simulink model "GFM_L_Filter_vc"  (R2019b)
settings: Solver=ode23tb  StartTime=0.0  StopTime=Simulation_Time  FixedStep=Time_Step2  MaxStep=1e-5  RelTol=1e-3
PreLoadFcn:
  | GFM_L_Filter_Init;
InitFcn:
  | GFM_L_Filter_Init;
undefined symbols (not defined in the file): Chosen_Strategy, DiscIntNeverNeededParam, dur1, dur2, egfault, fb, GRD00_Lg, GRD00_Lg2, GRD00_Rg, GRD00_Rg2, Ib2, Kc, kd, Ki_cc_cp, Ki_Inertia_Less, Kp_cc_cp, kp_GFo, Kp_Inertia_Less, R, Sb, SimStart, Theta_Vvsc0, Time_Step, Time_Step2, Ug, Va0, Vb0, Vb1, Vb2, Vc0, Vm0, VSC01_id0, Vvsc0, wb, Zb
libraries: powerlib x30, Control_Lib x15, simulink x7, Source_Lib x1, powerlib_meascontrol x1
(part 2 of 2)

== system GFM_L_Filter_vc/Generic Voltage Source/Source_For_OP ==
  v_abc_ref : Inport
  Controlled Voltage Source1 : powerlib/Electrical Sources/Controlled Voltage Source  Initialize=off  Source_Type=AC  Amplitude=V0*Ub*sqrt(2/3)*sin(Theta0)  Phase=(Theta0*180/pi)  Frequency=fb  Measurements=None
  Controlled Voltage Source2 : powerlib/Electrical Sources/Controlled Voltage Source  Initialize=off  Source_Type=AC  Amplitude=V0*Ub*sqrt(2/3)*sin(Theta0-2*pi/3)  Phase=(Theta0*180/pi)-120  Frequency=fb  Measurements=None
  Controlled Voltage Source3 : powerlib/Electrical Sources/Controlled Voltage Source  Initialize=off  Source_Type=AC  Amplitude=V0*Ub*sqrt(2/3)*sin(Theta0-4*pi/3)  Phase=(Theta0*180/pi)+120  Frequency=fb  Measurements=None
  Demux : Demux  Outputs=3
  Step : Step  Time=1e-9  SampleTime=0
  Subsystem3 : Subsystem
  Three-Phase Source1 : powerlib/Electrical Sources/Three-Phase Source  InternalConnection=Yn  VoltagePhases=off  Voltage=V0*Ub  PhaseAngle=Theta0  Voltage_phases=[25e3 25e3 25e3]/sqrt(3)  PhaseAngles_phases=[0 -120 +120]  Frequency=fb  NonIdealSource=off  SpecifyImpedance=off  Resistance=0.8929  Inductance=16.58e-3  ShortCircuitLevel=100e6  BaseVoltage=25e3  XRratio=7  BusType=swing  Pref=10e3  Qref=0  Prefabc=[10e3, 10e3, 10e3]  Qrefabc=[0, 0, 0]  Qmin=-inf  Qmax=inf
  A : PMIOPort  Side=Right
  B : PMIOPort  Port=2  Side=Right
  C : PMIOPort  Port=3  Side=Right
  N : PMIOPort  Port=4  Side=Left
  wires:
  Demux/2 -> Controlled Voltage Source2/1
  v_abc_ref/1 -> Demux/1
  Demux/1 -> Controlled Voltage Source1/1
  Demux/3 -> Controlled Voltage Source3/1
  Step/1 -> Subsystem3/1(switch)
  connections:
  Controlled Voltage Source3/LConn1 -- Three-Phase Source1/LConn1 -- N/RConn1 -- Controlled Voltage Source2/LConn1 -- Controlled Voltage Source1/LConn1
  Subsystem3/RConn1 -- A/RConn1
  Subsystem3/RConn2 -- B/RConn1
  Subsystem3/RConn3 -- C/RConn1
  Controlled Voltage Source1/RConn1 -- Subsystem3/LConn1
  Controlled Voltage Source2/RConn1 -- Subsystem3/LConn2
  Controlled Voltage Source3/RConn1 -- Subsystem3/LConn3
  Three-Phase Source1/RConn1 -- Subsystem3/LConn4
  Three-Phase Source1/RConn2 -- Subsystem3/LConn5
  Three-Phase Source1/RConn3 -- Subsystem3/LConn6

== system GFM_L_Filter_vc/GFM_VC_newwith_Pvirt IDEAL_VSC/Control loops2/ pu P//Q computation ==
  v_abc_pu : Inport  PortDimensions=3
  i_abc_pu : Inport  Port=2  PortDimensions=3
  Demux : Demux  Outputs=3
      settings: DisplayOption=none
  Mux : Mux  Inputs=3
  Product1 : Product  InputSameDT=on  SaturateOnIntegerOverflow=on  OutDataTypeStr=Inherit: Same as first input
  Product3 : Product  InputSameDT=on  SaturateOnIntegerOverflow=on  OutDataTypeStr=Inherit: Same as first input
  Sum : Sum  Inputs=+-  InputSameDT=on  SaturateOnIntegerOverflow=on  OutDataTypeStr=Inherit: Same as first input
  Sum1 : Sum  Inputs=1  InputSameDT=on  SaturateOnIntegerOverflow=on  OutDataTypeStr=Inherit: Same as first input
  Sum4 : Sum  Inputs=1  InputSameDT=on  SaturateOnIntegerOverflow=on  OutDataTypeStr=Inherit: Same as first input
  Sum5 : Sum  Inputs=+-  InputSameDT=on  SaturateOnIntegerOverflow=on  OutDataTypeStr=Inherit: Same as first input
  Sum6 : Sum  Inputs=+-  InputSameDT=on  SaturateOnIntegerOverflow=on  OutDataTypeStr=Inherit: Same as first input
  pu->V : Gain  Gain=1/sqrt(3)  SaturateOnIntegerOverflow=on  OutDataTypeStr=Inherit: Same as input  ParamDataTypeStr=Inherit: Same as input
  pu->V1 : Gain  Gain=1/3  SaturateOnIntegerOverflow=on  OutDataTypeStr=Inherit: Same as input  ParamDataTypeStr=Inherit: Same as input
  pu->V2 : Gain  Gain=1/3  SaturateOnIntegerOverflow=on  OutDataTypeStr=Inherit: Same as input  ParamDataTypeStr=Inherit: Same as input
  P : Outport  VectorParamsAs1DForOutWhenUnconnected=off
  Q : Outport  Port=2  VectorParamsAs1DForOutWhenUnconnected=off
  wires:
  pu->V2/1 -> Q/1
  pu->V1/1 -> P/1
  Sum1/1 -> pu->V/1
  Product3/1 -> Sum1/1
  Product1/1 -> Sum4/1
  v_abc_pu/1 -> Product1/1, Demux/1
  i_abc_pu/1 -> Product1/2, Product3/2
  Sum4/1 -> pu->V1/1
  Demux/1 -> Sum/1, Sum6/2
  Demux/2 -> Sum/2, Sum5/1
  Demux/3 -> Sum5/2, Sum6/1
  Sum/1 -> Mux/3
  Sum5/1 -> Mux/1
  Sum6/1 -> Mux/2
  Mux/1 -> Product3/1
  pu->V/1 -> pu->V2/1  "Q"

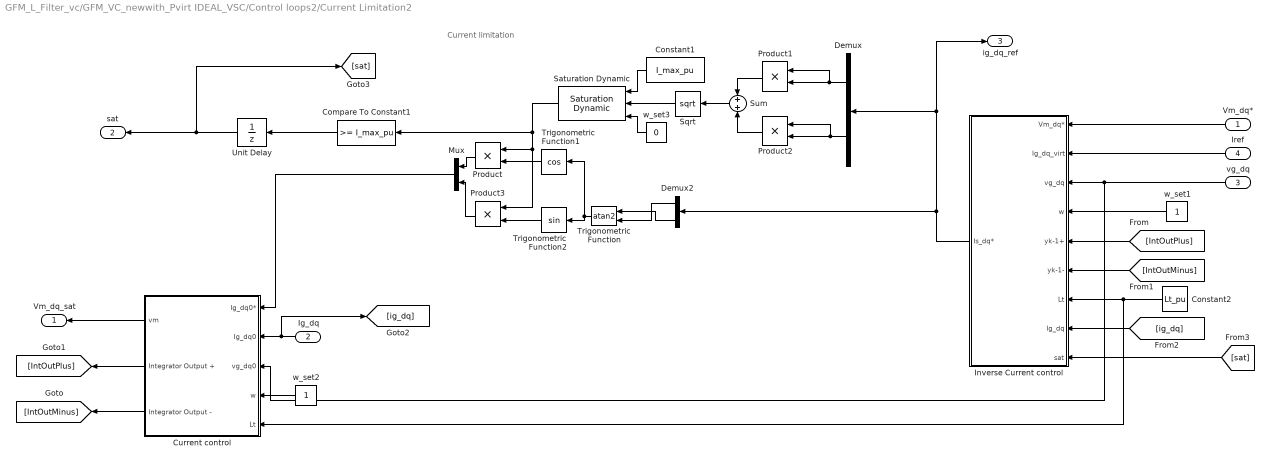
== system GFM_L_Filter_vc/GFM_VC_newwith_Pvirt IDEAL_VSC/Control loops2/Current Limitation2 ==
  note: Current limitation
  Vm_dq* : Inport
  Ig_dq : Inport  Port=2
  vg_dq : Inport  Port=3
  Iref : Inport  Port=4
  Compare To Constant1 : simulink/Logic and Bit Operations/Compare To Constant  relop=>=  const=I_max_pu  OutDataTypeStr=boolean
  Constant1 : Constant  Value=I_max_pu
  Constant2 : Constant  Value=Lt_pu
  Current control : Subsystem
  Demux : Demux  Outputs=2
  Demux2 : Demux  Outputs=2
  Inverse Current control : Subsystem
  Mux : Mux  Inputs=2
  Product{,1..3} (4 alike) : Product
  Saturation Dynamic : simulink/Discontinuities/Saturation Dynamic  OutMin=[]  OutMax=[]  OutDataTypeStr=Inherit: Same as second input  OutDataType=fixdt(1, 16)  OutScaling=2^-10  DoSatur=off
  Sqrt : Sqrt  SaturateOnIntegerOverflow=on
  Sum : Sum
  Trigonometric Function : Trigonometry  Operator=atan2  NumberOfIterations=5  OutputSignalType=real
  Trigonometric Function1 : Trigonometry  Operator=cos
  Trigonometric Function2 : Trigonometry
  Unit Delay : UnitDelay  SampleTime=-1  HasFrameUpgradeWarning=on
  w_set1 : Constant
  w_set2 : Constant
  w_set3 : Constant  Value=0
  Vm_dq_sat : Outport  VectorParamsAs1DForOutWhenUnconnected=off
  sat : Outport  Port=2
  ig_dq_ref : Outport  Port=3
  wires:
  w_set3/1 -> Saturation Dynamic/3
  Product/1 -> Mux/1
  Demux/1 -> Product1/1, Product1/2
  Demux/2 -> Product2/1, Product2/2
  Trigonometric Function2/1 -> Product3/2
  Product2/1 -> Sum/2
  Trigonometric Function1/1 -> Product/2
  Demux2/1 -> Trigonometric Function/2
  Trigonometric Function/1 -> Trigonometric Function2/1, Trigonometric Function1/1
  Product1/1 -> Sum/1
  Sqrt/1 -> Saturation Dynamic/2
  Demux2/2 -> Trigonometric Function/1
  Sum/1 -> Sqrt/1
  Product3/1 -> Mux/2
  Ig_dq/1 -> [ig_dq], Current control/2(Ig_dq0)
  w_set1/1 -> Inverse Current control/4(w)
  w_set2/1 -> Current control/4(w)
  Vm_dq*/1 -> Inverse Current control/1(Vm_dq*)
  Current control/1(vm) -> Vm_dq_sat/1
  Mux/1 -> Current control/1(Ig_dq0*)
  vg_dq/1 -> Current control/3(vg_dq0), Inverse Current control/3(vg_dq)
  Current control/3(Integrator Output -) -> [IntOutMinus]
  [IntOutMinus] -> Inverse Current control/6(yk-1-)
  Current control/2(Integrator Output +) -> [IntOutPlus]
  [IntOutPlus] -> Inverse Current control/5(yk-1+)
  Constant1/1 -> Saturation Dynamic/1
  Saturation Dynamic/1 -> Compare To Constant1/1, Product/1, Product3/1
  Compare To Constant1/1 -> Unit Delay/1
  Constant2/1 -> Current control/5(Lt), Inverse Current control/7(Lt)
  Iref/1 -> Inverse Current control/2(Ig_dq_virt)
  Inverse Current control/1(Is_dq*) -> Demux2/1, ig_dq_ref/1, Demux/1
  [ig_dq] -> Inverse Current control/8(Ig_dq)
  [sat] -> Inverse Current control/9(sat)
  Unit Delay/1 -> [sat], sat/1

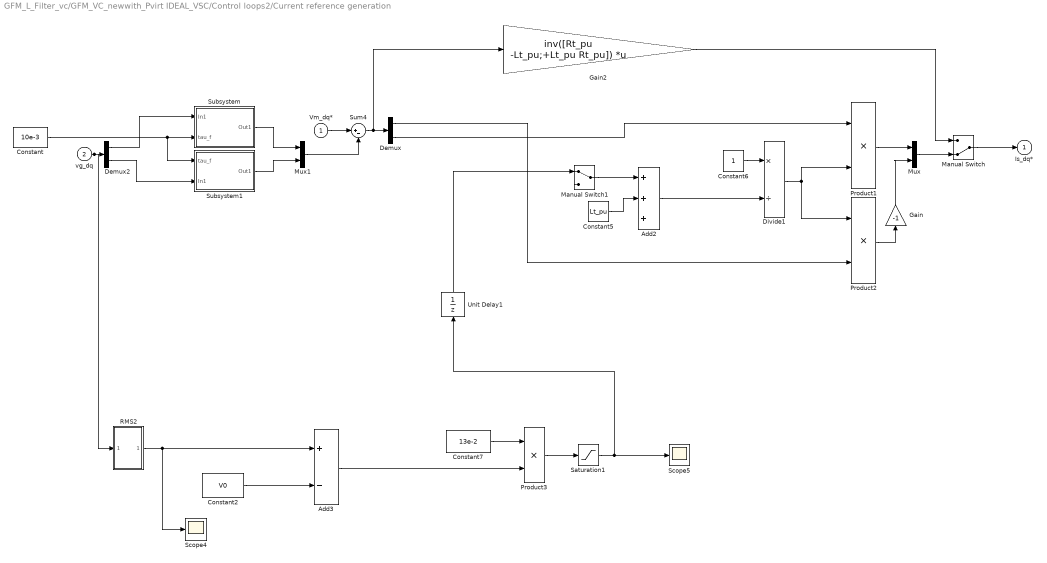
== system GFM_L_Filter_vc/GFM_VC_newwith_Pvirt IDEAL_VSC/Control loops2/Current reference generation ==
  Vm_dq* : Inport
  vg_dq : Inport  Port=2
  Add2 : Sum  Inputs=+++
  Add3 : Sum  Inputs=+-
  Constant : Constant  Value=10e-3
  Constant2 : Constant  Value=V0
  Constant5 : Constant  Value=Lt_pu
  Constant6 : Constant
  Constant7 : Constant  Value=13e-2
  Demux : Demux  Outputs=2
  Demux2 : Demux  Outputs=2
  Divide1 : Product  Inputs=*/
  Gain : Gain  Gain=-1
  Gain2 : Gain  Gain=inv([Rt_pu -Lt_pu;+Lt_pu Rt_pu])  Multiplication=Matrix(K*u)
  Manual Switch : ManualSwitch  CurrentSetting=0
  Manual Switch1 : ManualSwitch
  Mux : Mux  Inputs=2
  Mux1 : Mux  Inputs=2
  Product1 : Product
  Product2 : Product
  Product3 : Product
  RMS2 : Subsystem
  Saturation1 : Saturate  UpperLimit=0  LowerLimit=-0.14
  Scope4 : Scope
  Scope5 : Scope
  Subsystem : Subsystem
  Subsystem1 : Subsystem
  Sum4 : Sum  Inputs=|+-
  Unit Delay1 : UnitDelay  SampleTime=-1  HasFrameUpgradeWarning=on
  Is_dq* : Outport  InitialOutput=0  VectorParamsAs1DForOutWhenUnconnected=off
  wires:
  Unit Delay1/1 -> Manual Switch1/1
  Manual Switch1/1 -> Add2/1
  Vm_dq*/1 -> Sum4/1
  Demux2/2 -> Subsystem1/2(In1)
  Demux2/1 -> Subsystem/1(In1)
  Subsystem/1(Out1) -> Mux1/1
  Subsystem1/1(Out1) -> Mux1/2
  vg_dq/1 -> RMS2/1(Is_dq*), Demux2/1
  Sum4/1 -> Gain2/1, Demux/1
  Mux1/1 -> Sum4/2
  Constant/1 -> Subsystem1/1(tau_f), Subsystem/2(tau_f)
  Demux/2 -> Product1/1
  Product1/1 -> Mux/1
  Product2/1 -> Gain/1
  Demux/1 -> Product2/2
  Manual Switch/1 -> Is_dq*/1
  Gain2/1 -> Manual Switch/1
  Mux/1 -> Manual Switch/2
  Constant5/1 -> Add2/2
  Constant6/1 -> Divide1/1
  Divide1/1 -> Product2/1, Product1/2
  Gain/1 -> Mux/2
  Add2/1 -> Divide1/2
  Product3/1 -> Saturation1/1
  Constant2/1 -> Add3/2
  Constant7/1 -> Product3/1
  Add3/1 -> Product3/2
  RMS2/1(Out1) -> Add3/1, Scope4/1
  Saturation1/1 -> Unit Delay1/1, Scope5/1

== system GFM_L_Filter_vc/GFM_VC_newwith_Pvirt IDEAL_VSC/Control loops2/Power Control Loops1 ==
  P_mes : Inport
  P_set : Inport  Port=2
  delta_PLL : Inport  Port=3
  w_PLL : Inport  Port=4
  sat : Inport  Port=5
  Vg_rms : Inport  Port=6
  Compare To Constant : simulink/Logic and Bit Operations/Compare To Constant  relop===  const=1  OutDataTypeStr=boolean
  Compare To Constant1 : simulink/Logic and Bit Operations/Compare To Constant  relop===  const=2  OutDataTypeStr=boolean
  Compare To Constant2 : simulink/Logic and Bit Operations/Compare To Constant  relop===  const=3  OutDataTypeStr=boolean
  Inertia Less : Subsystem
  Multiport Switch : MultiPortSwitch
  Multiport Switch1 : MultiPortSwitch
  Mux : Mux  Inputs=[1 1]
  PI Controler : Subsystem
  Trigonometric Function : Trigonometry  Operator=cos
  Trigonometric Function1 : Trigonometry
  VSM : Subsystem
  w_set{1..4} (4 alike) : Constant  Value=Chosen_Strategy
  w_set_pu : Constant
  f : Outport  PortDimensions=1  VectorParamsAs1DForOutWhenUnconnected=off
  Theta : Outport  Port=2  VectorParamsAs1DForOutWhenUnconnected=off
  CosSinTheta : Outport  Port=3  PortDimensions=2  VectorParamsAs1DForOutWhenUnconnected=off
  wires:
  Trigonometric Function1/1 -> Mux/2
  Mux/1 -> CosSinTheta/1
  Trigonometric Function/1 -> Mux/1
  Compare To Constant2/1 -> PI Controler/Enable
  Compare To Constant1/1 -> VSM/Enable
  Compare To Constant/1 -> Inertia Less/Enable
  w_set4/1 -> Compare To Constant2/1
  w_set2/1 -> Compare To Constant1/1
  w_set3/1 -> Compare To Constant/1
  Inertia Less/1(frequency) -> Multiport Switch/2
  Multiport Switch/1 -> f/1
  Inertia Less/2(theta) -> Multiport Switch1/2
  VSM/2(theta) -> Multiport Switch1/3
  w_set1/1 -> Multiport Switch/1, Multiport Switch1/1
  VSM/1(frequency) -> Multiport Switch/3
  PI Controler/1(frequency) -> Multiport Switch/4
  PI Controler/2(theta) -> Multiport Switch1/4
  w_set_pu/1 -> PI Controler/3(w_set_pu)
  w_PLL/1 -> Inertia Less/4(w_PLL), VSM/3(w_PLL)
  delta_PLL/1 -> Inertia Less/3(delta_PLL)
  P_set/1 -> Inertia Less/2(P_set), VSM/2(P_set), PI Controler/2(P_set)
  P_mes/1 -> Inertia Less/1(P_mes), VSM/1(P_mes), PI Controler/1(P_mes)
  Multiport Switch1/1 -> Theta/1, Trigonometric Function1/1, Trigonometric Function/1
  sat/1 -> PI Controler/4(sat)
  Vg_rms/1 -> PI Controler/5(Vg_rms)

== system GFM_L_Filter_vc/GFM_VC_newwith_Pvirt IDEAL_VSC/Control loops2/Transient Damping Resistance ==
  ig_dq : Inport
  Filter w_LF : Subsystem
      mask Display: disp('\omega_{LF} / (s + \omega_{LF})','texmode','on')
  Sum5 : Sum  Inputs=|+-
  nq1 : Gain  Gain=Rv
  "Delta_E_dq " : Outport  VectorParamsAs1DForOutWhenUnconnected=off
  wires:
  nq1/1 -> Filter w_LF/1(e), Sum5/2
  Filter w_LF/1(s) -> Sum5/1
  Sum5/1 -> "Delta_E_dq "/1
  ig_dq/1 -> nq1/1

== system GFM_L_Filter_vc/GFM_VC_newwith_Pvirt IDEAL_VSC/Control loops2/Virtual Active Power calculation ==
  Voltage+ : Inport
  Current+ : Inport  Port=2
  Add2 : Sum
  Demux : Demux  Outputs=2
  Demux1 : Demux  Outputs=2
  Product : Product
  Product1 : Product
  Virtual Active Power : Outport
  wires:
  Product1/1 -> Add2/2
  Product/1 -> Add2/1
  Voltage+/1 -> Demux/1
  Current+/1 -> Demux1/1
  Demux/1 -> Product/2
  Demux/2 -> Product1/1
  Demux1/1 -> Product/1
  Demux1/2 -> Product1/2
  Add2/1 -> Virtual Active Power/1

== system GFM_L_Filter_vc/Generic Voltage Source/INERTIAL/CosSin ==
  Theta_rad : Inport
  Mux : Mux  Inputs=2
  Trigonometric Function : Trigonometry
  Trigonometric Function1 : Trigonometry  Operator=cos
  CosSinTheta : Outport  VectorParamsAs1DForOutWhenUnconnected=off
  wires:
  Trigonometric Function1/1 -> Mux/1
  Mux/1 -> CosSinTheta/1
  Trigonometric Function/1 -> Mux/2
  Theta_rad/1 -> Trigonometric Function1/1, Trigonometric Function/1

== system GFM_L_Filter_vc/Generic Voltage Source/INERTIAL/NetworkLeadLagTimeConstants ==
  In1 : Inport
  Constant : Constant  Value=P0
  Integrator3 : Integrator  InitialConditionSource=external  InitialCondition=(P0/Sb)*(1-TN/TD)
  Sum1 : Sum
  Sum2 : Sum  Inputs=+-
  Sum3 : Sum  Inputs=-+
  mp1 : Gain  Gain=TN/TD
  mp2 : Gain  Gain=1-TN/TD
  mp3 : Gain  Gain=1/TD
  Out1 : Outport  VectorParamsAs1DForOutWhenUnconnected=off
  wires:
  Sum3/1 -> Integrator3/2
  Integrator3/1 -> Sum2/2, Sum1/2
  Constant/1 -> Sum3/2
  Sum2/1 -> mp3/1
  mp3/1 -> Integrator3/1
  In1/1 -> mp1/1, mp2/1
  mp2/1 -> Sum2/1
  mp1/1 -> Sum1/1, Sum3/1
  Sum1/1 -> Out1/1

== system GFM_L_Filter_vc/Generic Voltage Source/INFINITE/CosSin ==
  Theta_rad : Inport
  Mux : Mux  Inputs=2
  Trigonometric Function : Trigonometry
  Trigonometric Function1 : Trigonometry  Operator=cos
  CosSinTheta : Outport  VectorParamsAs1DForOutWhenUnconnected=off
  wires:
  Trigonometric Function1/1 -> Mux/1
  Mux/1 -> CosSinTheta/1
  Trigonometric Function/1 -> Mux/2
  Theta_rad/1 -> Trigonometric Function1/1, Trigonometric Function/1

== system GFM_L_Filter_vc/Generic Voltage Source/Source_For_OP/Subsystem3 ==
  switch : Inport
  Breaker : powerlib/Elements/Breaker  InitialState=0  SwitchingTimes="[1/60  5/60]"  External=on  BreakerResistance=0.001  SnubberResistance=1e6  SnubberCapacitance=inf  Measurements=None  MoreParameters=on  NoBreakLoop=off
  Breaker1 : powerlib/Elements/Breaker  InitialState=0  SwitchingTimes="[1/60  5/60]"  External=on  BreakerResistance=0.001  SnubberResistance=1e6  SnubberCapacitance=inf  Measurements=None  MoreParameters=on  NoBreakLoop=off
  Breaker2 : powerlib/Elements/Breaker  InitialState=0  SwitchingTimes="[1/60  5/60]"  External=on  BreakerResistance=0.001  SnubberResistance=1e6  SnubberCapacitance=inf  Measurements=None  MoreParameters=on  NoBreakLoop=off
  Breaker3 : powerlib/Elements/Breaker  InitialState=1  SwitchingTimes="[1/60  5/60]"  External=on  BreakerResistance=0.001  SnubberResistance=1e6  SnubberCapacitance=inf  Measurements=None  MoreParameters=on  NoBreakLoop=off
  Breaker4 : powerlib/Elements/Breaker  InitialState=1  SwitchingTimes="[1/60  5/60]"  External=on  BreakerResistance=0.001  SnubberResistance=1e6  SnubberCapacitance=inf  Measurements=None  MoreParameters=on  NoBreakLoop=off
  Breaker5 : powerlib/Elements/Breaker  InitialState=1  SwitchingTimes="[1/60  5/60]"  External=on  BreakerResistance=0.001  SnubberResistance=1e6  SnubberCapacitance=inf  Measurements=None  MoreParameters=on  NoBreakLoop=off
  Logical Operator : Logic  Operator=NOT  AllPortsSameDT=off  OutDataTypeStr=boolean
  A : PMIOPort  Side=Left
  B : PMIOPort  Port=2  Side=Left
  C : PMIOPort  Port=3  Side=Left
  Ainit : PMIOPort  Port=4  Side=Left
  Binit : PMIOPort  Port=5  Side=Left
  Cinit : PMIOPort  Port=6  Side=Left
  a : PMIOPort  Port=7  Side=Right
  b : PMIOPort  Port=8  Side=Right
  c : PMIOPort  Port=9  Side=Right
  wires:
  switch/1 -> Breaker2/1, Breaker1/1, Breaker/1, Logical Operator/1
  Logical Operator/1 -> Breaker5/1, Breaker4/1, Breaker3/1
  connections:
  Breaker/LConn1 -- A/RConn1
  Breaker5/LConn1 -- Cinit/RConn1
  c/RConn1 -- Breaker5/RConn1 -- Breaker2/RConn1
  Breaker4/LConn1 -- Binit/RConn1
  Breaker2/LConn1 -- C/RConn1
  Breaker3/LConn1 -- Ainit/RConn1
  Breaker1/LConn1 -- B/RConn1
  Breaker/RConn1 -- Breaker3/RConn1 -- a/RConn1
  b/RConn1 -- Breaker1/RConn1 -- Breaker4/RConn1

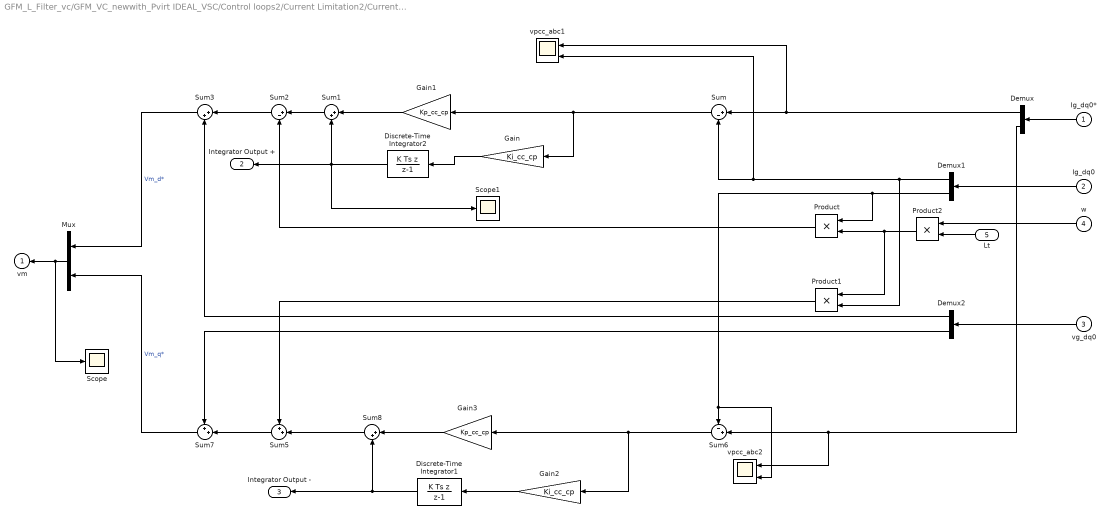
== system GFM_L_Filter_vc/GFM_VC_newwith_Pvirt IDEAL_VSC/Control loops2/Current Limitation2/Current control ==
  Ig_dq0* : Inport
  Ig_dq0 : Inport  Port=2
  vg_dq0 : Inport  Port=3
  w : Inport  Port=4
  Lt : Inport  Port=5
  Demux : Demux  Outputs=2
  Demux1 : Demux  Outputs=2
  Demux2 : Demux  Outputs=2
  Discrete-Time Integrator1 : DiscreteIntegrator  IntegratorMethod=Integration: Backward Euler  SampleTime=Output_Delay  ICPrevOutput=DiscIntNeverNeededParam  ICPrevScaledInput=DiscIntNeverNeededParam
  Discrete-Time Integrator2 : DiscreteIntegrator  IntegratorMethod=Integration: Backward Euler  SampleTime=Output_Delay  ICPrevOutput=DiscIntNeverNeededParam  ICPrevScaledInput=DiscIntNeverNeededParam
  Gain : Gain  Gain=Ki_cc_cp
  Gain1 : Gain  Gain=Kp_cc_cp
  Gain2 : Gain  Gain=Ki_cc_cp
  Gain3 : Gain  Gain=Kp_cc_cp
  Mux : Mux  Inputs=2
  Product : Product  RndMeth=Zero
  Product1 : Product  RndMeth=Zero
  Product2 : Product  RndMeth=Zero
  Scope : Scope
  Scope1 : Scope
  Sum : Sum  Inputs=|+-
  Sum1 : Sum  Inputs=|++
  Sum2 : Sum  Inputs=|+-
  Sum3 : Sum  Inputs=|++
  Sum5 : Sum  Inputs=++|
  Sum6 : Sum  Inputs=-+|
  Sum7 : Sum  Inputs=++|
  Sum8 : Sum  Inputs=|++
  vpcc_abc1 : Scope  NumInputPorts=2
  vpcc_abc2 : Scope  NumInputPorts=2
  vm : Outport  InitialOutput=0  VectorParamsAs1DForOutWhenUnconnected=off
  Integrator Output + : Outport  Port=2
  Integrator Output - : Outport  Port=3
  wires:
  w/1 -> Product2/1
  Sum/1 -> Gain/1, Gain1/1
  Sum7/1 -> Mux/2  "Vm_q*"
  Sum3/1 -> Mux/1  "Vm_d*"
  Sum5/1 -> Sum7/2
  Product1/1 -> Sum5/1
  Demux/2 -> vpcc_abc2/1, Sum6/2
  Sum2/1 -> Sum3/1
  Product/1 -> Sum2/2
  Product2/1 -> Product1/1, Product/2
  Demux1/1 -> vpcc_abc1/2, Sum/2, Product1/2
  Ig_dq0/1 -> Demux1/1
  vg_dq0/1 -> Demux2/1
  Ig_dq0*/1 -> Demux/1
  Mux/1 -> Scope/1, vm/1
  Demux1/2 -> vpcc_abc2/2, Sum6/1, Product/1
  Demux2/1 -> Sum3/2
  Sum1/1 -> Sum2/1
  Sum8/1 -> Sum5/2
  Demux2/2 -> Sum7/1
  Gain/1 -> Discrete-Time Integrator2/1
  Gain1/1 -> Sum1/1
  Gain3/1 -> Sum8/1
  Gain2/1 -> Discrete-Time Integrator1/1
  Sum6/1 -> Gain2/1, Gain3/1
  Discrete-Time Integrator1/1 -> Sum8/2, Integrator Output -/1
  Lt/1 -> Product2/2
  Demux/1 -> vpcc_abc1/1, Sum/1
  Discrete-Time Integrator2/1 -> Integrator Output +/1, Scope1/1, Sum1/2

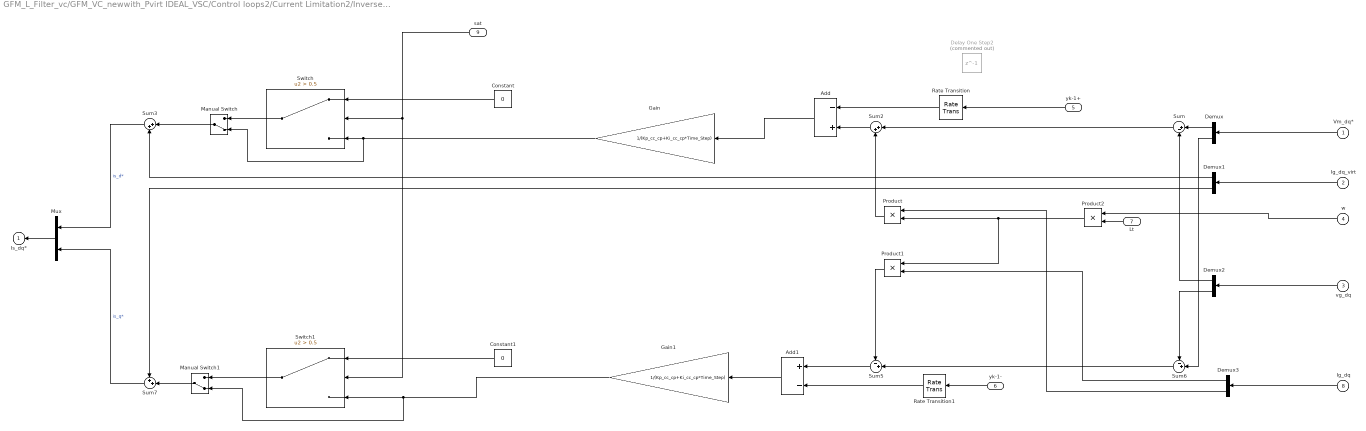
== system GFM_L_Filter_vc/GFM_VC_newwith_Pvirt IDEAL_VSC/Control loops2/Current Limitation2/Inverse Current control ==
  Vm_dq* : Inport
  Ig_dq_virt : Inport  Port=2
  vg_dq : Inport  Port=3
  w : Inport  Port=4
  yk-1+ : Inport  Port=5
  yk-1- : Inport  Port=6
  Lt : Inport  Port=7
  Ig_dq : Inport  Port=8
  sat : Inport  Port=9
  Add : Sum  Inputs=-+
  Add1 : Sum  Inputs=+-
  Constant : Constant  Value=0
  Constant1 : Constant  Value=0
  Delay One Step2 : Delay  Commented=on  DelayLength=1  SampleTime=Time_Step
  Demux{,1..3} (4 alike) : Demux  Outputs=2
  Gain : Gain  Gain=1/(Kp_cc_cp+Ki_cc_cp*Time_Step)
  Gain1 : Gain  Gain=1/(Kp_cc_cp+Ki_cc_cp*Time_Step)
  Manual Switch : ManualSwitch  CurrentSetting=0
  Manual Switch1 : ManualSwitch  CurrentSetting=0
  Mux : Mux  Inputs=2
  Product : Product  RndMeth=Zero
  Product1 : Product  RndMeth=Zero
  Product2 : Product
  Rate Transition : RateTransition  OutPortSampleTime=Output_Delay
  Rate Transition1 : RateTransition  OutPortSampleTime=Output_Delay
  Sum : Sum  Inputs=|+-
  Sum2 : Sum  Inputs=|++
  Sum3 : Sum  Inputs=|++
  Sum5 : Sum  Inputs=-+|
  Sum6 : Sum  Inputs=-+|
  Sum7 : Sum  Inputs=++|
  Switch : Switch  Criteria=u2 > Threshold  Threshold=0.5
  Switch1 : Switch  Criteria=u2 > Threshold  Threshold=0.5
  Is_dq* : Outport  InitialOutput=0  VectorParamsAs1DForOutWhenUnconnected=off
  wires:
  Ig_dq_virt/1 -> Demux1/1
  Vm_dq*/1 -> Demux/1
  Demux/1 -> Sum/1
  Demux1/1 -> Sum3/2
  Sum/1 -> Sum2/1
  Product2/1 -> Product1/1, Product/2
  Sum2/1 -> Add/2
  Mux/1 -> Is_dq*/1
  Demux/2 -> Sum6/2
  Sum6/1 -> Sum5/2
  Sum3/1 -> Mux/1  "is_d*"
  Sum7/1 -> Mux/2  "is_q*"
  w/1 -> Product2/1
  Demux1/2 -> Sum7/1
  yk-1+/1 -> Rate Transition/1
  Rate Transition/1 -> Add/1
  Add/1 -> Gain/1
  Add1/1 -> Gain1/1
  Sum5/1 -> Add1/1
  yk-1-/1 -> Rate Transition1/1
  Rate Transition1/1 -> Add1/2
  Product1/1 -> Sum5/1
  Product/1 -> Sum2/2
  vg_dq/1 -> Demux2/1
  Demux2/2 -> Sum6/1
  Demux2/1 -> Sum/2
  Lt/1 -> Product2/2
  Ig_dq/1 -> Demux3/1
  Demux3/2 -> Product/1
  Demux3/1 -> Product1/2
  sat/1 -> Switch1/2, Switch/2
  Gain/1 -> Manual Switch/2, Switch/3
  Constant/1 -> Switch/1
  Constant1/1 -> Switch1/1
  Gain1/1 -> Manual Switch1/2, Switch1/3
  Manual Switch/1 -> Sum3/1
  Switch/1 -> Manual Switch/1
  Manual Switch1/1 -> Sum7/2
  Switch1/1 -> Manual Switch1/1

== system GFM_L_Filter_vc/GFM_VC_newwith_Pvirt IDEAL_VSC/Control loops2/Current reference generation/RMS2 ==
  Is_dq* : Inport
  Demux : Demux  Outputs=2
  Sqrt : Sqrt  SaturateOnIntegerOverflow=on
  Square : Math  Operator=square  SaturateOnIntegerOverflow=on
  Square1 : Math  Operator=square  SaturateOnIntegerOverflow=on
  Sum : Sum  Inputs=|++
  Out1 : Outport
  wires:
  Demux/2 -> Square1/1
  Is_dq*/1 -> Demux/1
  Demux/1 -> Square/1
  Sqrt/1 -> Out1/1
  Square1/1 -> Sum/2
  Square/1 -> Sum/1
  Sum/1 -> Sqrt/1

== system GFM_L_Filter_vc/GFM_VC_newwith_Pvirt IDEAL_VSC/Control loops2/Current reference generation/Subsystem ==
  In1 : Inport
  tau_f : Inport  Port=2
  Integrator : Integrator  InitialConditionSource=external  InitialCondition=1
  Product : Product  Inputs=/*
  Sum2 : Sum  Inputs=|+-
  Out1 : Outport
  wires:
  Product/1 -> Integrator/1
  Sum2/1 -> Product/2
  Integrator/1 -> Sum2/2, Out1/1
  tau_f/1 -> Product/1
  In1/1 -> Integrator/2, Sum2/1

== system GFM_L_Filter_vc/GFM_VC_newwith_Pvirt IDEAL_VSC/Control loops2/Current reference generation/Subsystem1 ==
  tau_f : Inport
  In1 : Inport  Port=2
  Integrator : Integrator  InitialConditionSource=external
  Product : Product  Inputs=/*
  Sum2 : Sum  Inputs=|+-
  Out1 : Outport
  wires:
  Product/1 -> Integrator/1
  Sum2/1 -> Product/2
  Integrator/1 -> Sum2/2, Out1/1
  In1/1 -> Sum2/1, Integrator/2
  tau_f/1 -> Product/1

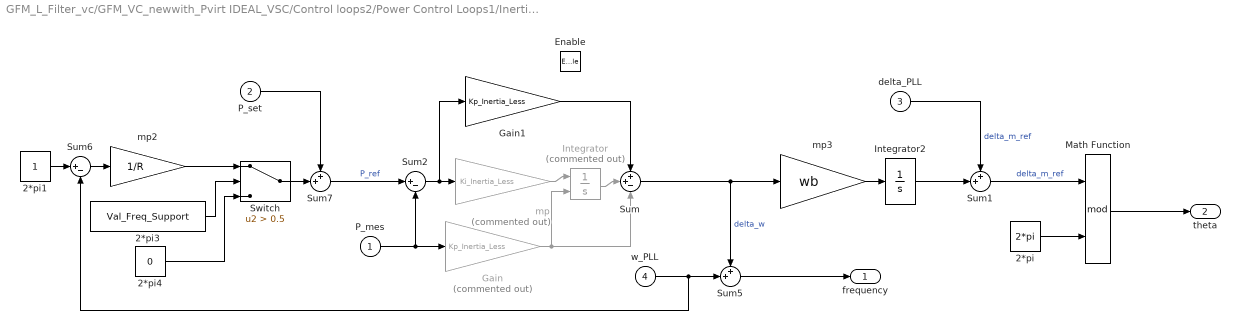
== system GFM_L_Filter_vc/GFM_VC_newwith_Pvirt IDEAL_VSC/Control loops2/Power Control Loops1/Inertia Less ==
  P_mes : Inport
  P_set : Inport  Port=2
  delta_PLL : Inport  Port=3
  w_PLL : Inport  Port=4
  Enable : EnablePort
  2*pi : Constant  Value=2*pi
  2*pi1 : Constant
  2*pi3 : Constant  Value=Val_Freq_Support
  2*pi4 : Constant  Value=0
  Gain : Gain  Commented=on  Gain=Kp_Inertia_Less
  Gain1 : Gain  Gain=Kp_Inertia_Less
  Integrator : Integrator  Commented=on  InitialConditionSource=external
  Integrator2 : Integrator  InitialCondition=(Theta0_VSC)*pi/180-Theta0*pi/180
  Math Function : Math  Operator=mod  SignedPower=on  SaturateOnIntegerOverflow=on
  Sum : Sum  Inputs=++-
  Sum1 : Sum  Inputs=++|
  Sum2 : Sum  Inputs=|+-
  Sum5 : Sum  Inputs=++|
  Sum6 : Sum  Inputs=|+-
  Sum7 : Sum  Inputs=++|
  Switch : Switch  Criteria=u2 > Threshold  Threshold=0.5
  mp : Gain  Commented=on  Gain=Ki_Inertia_Less
  mp2 : Gain  Gain=1/R
  mp3 : Gain  Gain=wb
  frequency : Outport  VectorParamsAs1DForOutWhenUnconnected=off
  theta : Outport  Port=2  VectorParamsAs1DForOutWhenUnconnected=off
  wires:
  Sum5/1 -> frequency/1
  Switch/1 -> Sum7/2
  Gain1/1 -> Sum/1
  Gain/1 -> Integrator/2, Sum/3
  Integrator/1 -> Sum/2
  2*pi4/1 -> Switch/3
  2*pi3/1 -> Switch/2
  mp2/1 -> Switch/1
  Integrator2/1 -> Sum1/2
  w_PLL/1 -> Sum5/2, Sum6/2
  delta_PLL/1 -> Sum1/1  "delta_m_ref"
  mp/1 -> Integrator/1
  mp3/1 -> Integrator2/1
  Sum/1 -> mp3/1, Sum5/1  "delta_w"
  Math Function/1 -> theta/1
  P_mes/1 -> Sum2/2, Gain/1
  Sum7/1 -> Sum2/1  "P_ref"
  P_set/1 -> Sum7/1
  Sum6/1 -> mp2/1
  2*pi1/1 -> Sum6/1
  2*pi/1 -> Math Function/2
  Sum1/1 -> Math Function/1  "delta_m_ref"
  Sum2/1 -> mp/1, Gain1/1

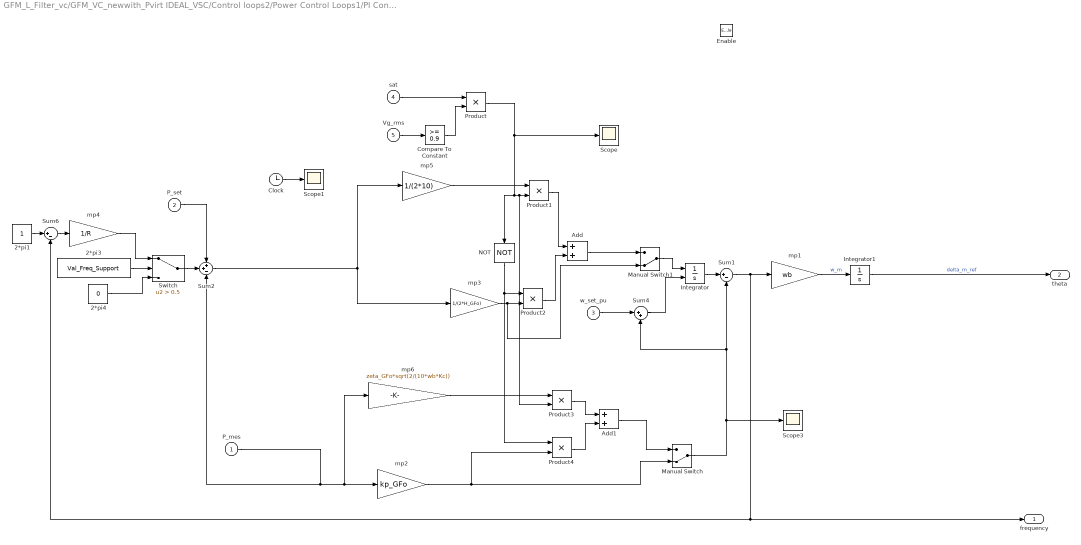
== system GFM_L_Filter_vc/GFM_VC_newwith_Pvirt IDEAL_VSC/Control loops2/Power Control Loops1/PI Controler ==
  P_mes : Inport
  P_set : Inport  Port=2
  w_set_pu : Inport  Port=3
  sat : Inport  Port=4
  Vg_rms : Inport  Port=5
  Enable : EnablePort
  2*pi1 : Constant
  2*pi3 : Constant  Value=Val_Freq_Support
  2*pi4 : Constant  Value=0
  Add : Sum
  Add1 : Sum
  Clock : Clock
  Compare To Constant : simulink/Logic and Bit Operations/Compare To Constant  relop=>=  const=0.9  OutDataTypeStr=boolean
  Integrator : Integrator  InitialConditionSource=external
  Integrator1 : Integrator  InitialCondition=(Theta0_VSC)*pi/180
  Manual Switch : ManualSwitch  CurrentSetting=0
  Manual Switch1 : ManualSwitch  CurrentSetting=0
  NOT : Logic  Operator=NOT  IconShape=distinctive  AllPortsSameDT=off  OutDataTypeStr=boolean
  Product{,1..4} (5 alike) : Product
  Scope : Scope
  Scope1 : Scope
  Scope3 : Scope
  Sum1 : Sum  Inputs=|+-
  Sum2 : Sum  Inputs=++-
  Sum4 : Sum  Inputs=|++
  Sum6 : Sum  Inputs=|+-
  Switch : Switch  Criteria=u2 > Threshold  Threshold=0.5
  mp1 : Gain  Gain=wb
  mp2 : Gain  Gain=kp_GFo
  mp3 : Gain  Gain=1/(2*H_GFo)
  mp4 : Gain  Gain=1/R
  mp5 : Gain  Gain=1/(2*10)
  mp6 : Gain  Gain=zeta_GFo*sqrt(2/(10*wb*Kc))
  frequency : Outport  VectorParamsAs1DForOutWhenUnconnected=off
  theta : Outport  Port=2  VectorParamsAs1DForOutWhenUnconnected=off
  wires:
  Switch/1 -> Sum2/2
  2*pi4/1 -> Switch/3
  Sum6/1 -> mp4/1
  2*pi3/1 -> Switch/2
  2*pi1/1 -> Sum6/1
  mp4/1 -> Switch/1
  Sum4/1 -> Integrator/2
  P_mes/1 -> Sum2/3, mp6/1, mp2/1
  mp1/1 -> Integrator1/1  "w_m"
  Sum1/1 -> Sum6/2, frequency/1, mp1/1
  Integrator/1 -> Sum1/1
  P_set/1 -> Sum2/1
  w_set_pu/1 -> Sum4/1
  Integrator1/1 -> theta/1  "delta_m_ref"
  Sum2/1 -> mp3/1, mp5/1
  Vg_rms/1 -> Compare To Constant/1
  sat/1 -> Product/1
  Compare To Constant/1 -> Product/2
  mp6/1 -> Product3/1
  mp2/1 -> Product4/2, Manual Switch/2
  Clock/1 -> Scope1/1
  Add1/1 -> Manual Switch/1
  Manual Switch/1 -> Scope3/1, Sum1/2, Sum4/2
  Manual Switch1/1 -> Integrator/1
  mp5/1 -> Product1/1
  Product/1 -> Scope/1, Product3/2, Product1/2, NOT/1
  Product1/1 -> Add/1
  NOT/1 -> Product4/1, Product2/1
  Product2/1 -> Add/2
  Add/1 -> Manual Switch1/1
  mp3/1 -> Manual Switch1/2, Product2/2
  Product3/1 -> Add1/1
  Product4/1 -> Add1/2

== system GFM_L_Filter_vc/GFM_VC_newwith_Pvirt IDEAL_VSC/Control loops2/Power Control Loops1/VSM ==
  P_mes : Inport
  P_set : Inport  Port=2
  w_PLL : Inport  Port=3
  Enable : EnablePort
  2*pi1 : Constant
  2*pi3 : Constant  Value=Val_Freq_Support
  2*pi4 : Constant  Value=0
  Gain : Gain  Gain=kd
  Gain1 : Gain  Gain=1/(2*H_GFo)
  Integrator : Integrator  InitialCondition=1
  Integrator1 : Integrator  InitialCondition=Theta0_VSC*pi/180
  Sum : Sum  Inputs=|+-
  Sum1 : Sum  Inputs=++-
  Sum6 : Sum  Inputs=|+-
  Sum7 : Sum  Inputs=++|
  Switch : Switch  Criteria=u2 > Threshold  Threshold=0.5
  mp1 : Gain  Gain=1/R
  mp2 : Gain  Gain=wb
  frequency : Outport  VectorParamsAs1DForOutWhenUnconnected=off
  theta : Outport  Port=2  VectorParamsAs1DForOutWhenUnconnected=off
  wires:
  Gain1/1 -> Integrator/1
  Sum7/1 -> Sum1/2  "P_ref"
  Sum1/1 -> Gain1/1
  Gain/1 -> Sum1/1
  Sum/1 -> Gain/1
  w_PLL/1 -> Sum/1
  2*pi4/1 -> Switch/3
  2*pi3/1 -> Switch/2
  mp1/1 -> Switch/1
  2*pi1/1 -> Sum6/1
  Sum6/1 -> mp1/1
  P_set/1 -> Sum7/1
  Switch/1 -> Sum7/2
  mp2/1 -> Integrator1/1
  P_mes/1 -> Sum1/3
  Integrator/1 -> Sum6/2, frequency/1, mp2/1, Sum/2  "wm"
  Integrator1/1 -> theta/1  "delta_m_ref"

== system GFM_L_Filter_vc/GFM_VC_newwith_Pvirt IDEAL_VSC/Control loops2/Transient Damping Resistance/Filter w_LF ==
  e : Inport
  1/T_LP : Gain  Gain=W_TVR  SaturateOnIntegerOverflow=on  OutDataTypeStr=Inherit: Same as input  ParamDataTypeStr=Inherit: Same as input
  Integrator : Integrator  InitialConditionSource=external  InitialCondition=[VSC01_id0*0.04]
  Sum1 : Sum  Inputs=|+-  InputSameDT=on  SaturateOnIntegerOverflow=on  OutDataTypeStr=Inherit: Same as first input
  s : Outport  VectorParamsAs1DForOutWhenUnconnected=off
  wires:
  e/1 -> Sum1/1, Integrator/2
  Integrator/1 -> s/1, Sum1/2
  1/T_LP/1 -> Integrator/1
  Sum1/1 -> 1/T_LP/1
